simulink model "ava2"  (R2017b)
settings: Solver=VariableStepAuto  StartTime=0.0  StopTime=10.0  RelTol=1e-3
model workspace (MAT data in the model file):
  env_Snm = [1; 1; 1.5; 1.73205080757; 0.866025403784; 2.5; 3.06186217848; 1.9364916731; 0.790569415042; 4.375; 5.53398590529; 3.91311896062; 2.09165006634; 0.739509972887; 7.875; 10.1665812838; 7.68521307447; 4.70621264925; 2.21852991866; 0.70156076002; 14.4375; 18.9031247417; 14.9442322695; 9.96282151301; 5.45686207907; 2.32681380862; 0.671693289381; 26.8125; 35.469603514; 28.960809996; 20.4783851368; 12.3489308748; 6.17446543739; 2.42182459625; 0.647259849288; 50.2734375; 67.03125; 56.0823674036; 41.4195733282; 26.7362196178; 14.8305862683; 6.86522742932; 2.50682661696; 0.62670665424; 94.9609375; 127.403466874; 108.650041615; 82.9828399936; 56.3757383717; 33.6909476871; 17.3979305747; 7.53352492547; 2.58397773171; 0.609049392176; 180.42578125; 243.286073807; 210.691920304; 165.280340459; 116.870849536; 73.9156153223; 41.3200851149; 20.0431853398; 8.18259615041; 2.65478475212; 0.593627917137; 344.44921875; 466.386446929; 409.047973375; 327.968008098; 239.513968234; 158.423598868; 94.1176423013; 49.6043529462; 22.7600380686; 8.81492483989; 2.72034486492; 0.579979473935; 660.194335938; 897.027461585; 795.129860697; 649.220812653; 486.91560949; 334.021352445; 208.298910119; 117.053882271; 58.5269411357; 25.5432512332; 9.43247063627; 2.78148384397; 0.567768012127]
  env_WMMGC = [1 1 2 2 2 3 3 3 3 4 4 4 ... (540 elements, 90x6)]
settings Model: Creator=hbourbou  LastModifiedBy=hbourbou

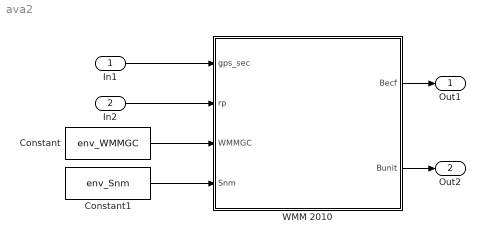
== system ava2 ==
  In1 : Inport
  In2 : Inport  Port=2  PortDimensions=3
  Constant : Constant  Value=env_WMMGC
  Constant1 : Constant  Value=env_Snm
  WMM 2010 : MATLAB Function  TreatAsAtomicUnit=on
  Out1 : Outport
  Out2 : Outport  Port=2
  wires:
  In1/1 -> WMM 2010/1(gps_sec)
  In2/1 -> WMM 2010/2(rp)
  Constant/1 -> WMM 2010/3(WMMGC)
  Constant1/1 -> WMM 2010/4(Snm)
  WMM 2010/1(Becf) -> Out1/1
  WMM 2010/2(Bunit) -> Out2/1

== matlab function ava2/WMM 2010 ==
  data: gps_sec input; Becf output; rp input; WMMGC input; Snm input; Bunit output
%% World Magnetic Model (Valid until Dec 31 2015, needs coefficient update and leap year compesation after this date)
% Requires file magm.m

%% Code
function [Becf, Bunit] = fcn(gps_sec,rp, WMMGC, Snm)


[Becf,Bunit]= magm(rp,gps_sec, WMMGC, Snm);

end

function [Becf,Bunit]=magm(rp,gps_sec,WMMGC, Snm)
%#codegen
% This function computes the magnetic field vector at a given position in space
% Note: altitude limited to 850km above the geomagnetic referemce radius (6371.2 km)

% Vivek Nagabhushan
% May 31 2013le
% Millenium Engineering and Integration Company
% Revised 02/12/2018 Sonny - Model(i.e. WMMGC, snm) is valid through 01/01/2020

% Inputs: Schmidt normalized WMM Gaussian coefficients, position vector in
% the form rp=[phi_gd lambda h_ellp] where, h_ellp is the height above the WGS-84 ellipsoid in kilometers, phi_gd is
% the geodetic latitude in degrees, and lambda is the East longitude from the Greenwich meridian in degrees

% Output: Unit magnetic field vector in ECEF coordinates. Other output forms
% can be chosen if desired

% Other files: index.m, coeffcnvrt.m, R_ECF_NED.m, WMMGC.mat, and Snm.mat

% References:
% 1. Maus, S., S. Macmillan, S. McLean, B. Hamilton, A. Thomson, M. Nair, and C. Rollins, 2010, The US/UK World Magnetic Model for 2010-2015
% 2. Plett, M., 'Magnetic Models' in 'Spacecraft Attitude Determination and Control', Edited by Wertz, J., Kluwer Academic Publishers, 1990
% 3. Davis, J., 'Mathematical Modeling of Earth's Magnetic Field', Technical Note, 'http://hanspeterschaub.info/Papers/UnderGradStudents/MagneticField.pdf', 2004
% 4. Notation for latitude and longitude consistent with Vallado, D. A., 'Fundamentals of Astrodynamics and Applications', 4th Edition, Space Technology Library, 2013

%years since 2015-01-01-00:00:00
% seconds between 2015-01-01-00:00:00 and 1980-01-06:00:00:00 = 1104105616
wmm_sec = gps_sec - 1104105616;
years   = wmm_sec/60/60/24/365;
if(gps_sec > 1140739217) %then leap day has occured!
    years = years + 1/365;
end


r_mag=6371.200; % Geomagnetic reference radius of the Earth in kilometers
Re=6378.137; % Semi-major axis of the Earth ellipsoid / Earth Equatorial radius in kilometers
esquared=0.006694379990141; % Eccentricity that models the Earth oblateness
[g,h]=coeffcnvrt(years, WMMGC, Snm); % Returns Schmidt normalized Gaussian coefficients


phi_gd=rp(1)*pi/180; % Geodetic Latitude
lambda=rp(2)*pi/180; % Geodetic Longitude = Geocentric Longitude
h_ellp=rp(3); % Height above the reference ellipsoid in kilometers (The height reported by GPS is the height above ellipsoid or HAE. The ellipsoid is the WGS84 )

% Convert Geodetic coordinates to Geocentric 
C=Re/sqrt(1-esquared*sin(phi_gd)^2);
rd=(C+h_ellp)*cos(phi_gd);
rk=(C*(1-esquared)+h_ellp)*sin(phi_gd);
r=sqrt(rd^2+rk^2); % Geocentric distance
phi_gc=asin(rk/r); % Conversion from Geodetic Latitude to Geocentric Latitude
co_phi_gc=(pi/2)-phi_gc; % Conversion from latitude to co-latitude
s=sin(co_phi_gc);
c=cos(co_phi_gc);
cl=cos(lambda);
sl=sin(lambda);

K=zeros(90,1);
P=zeros(90,1);
dP=zeros(90,1);
Br=0; 
Bp=0; %B_phi
Bl=0; %B_lambda


% Compute coefficients K and Gaussian-normalized associated Legendre functions, Pnm

P(1)=c;
P(2)=s;
P(3)=c^2-0.33333;
P(4)=c*s;
P(5)=s^2;
dP(1)=-s;
dP(2)=c;
dP(3)=-2*s*c;
dP(4)=c^2-s^2;
dP(5)=2*s*c;


for n=3:12 % Note that values of the fucntions for n=1,2 have been precomputed so that the case of index(0,0) is not encountered
    for m=0:n
        
        if m==n
            P(index(n,m))=s*P(index(n-1,m-1));
            dP(index(n,m))=s*dP(index(n-1,m-1))+c*P(index(n-1,m-1));
        else
            if m>(n-2)
                Pnm2=0;
                dPnm2=0;
            else
                Pnm2=P(index(n-2,m));
                dPnm2=dP(index(n-2,m));
            end
            
            K(index(n,m))=((n-1)^2-m^2)/((2*n-1)*(2*n-3)); % Note that K(1,1) and K(1,0) are equal to zero
            P(index(n,m))=c*P(index(n-1,m))-K(index(n,m))*Pnm2;
            dP(index(n,m))=c*dP(index(n-1,m))-s*P(index(n-1,m))-K(index(n,m))*dPnm2;
        end
               
    end
end


% Spherical coordinate components (Br,B_phi,B_lambda) of magnetic field

cml=0;sml=0;cmm1l=0;smm1l=0; % Initialize to avoid error in Simulink

for n=1:12
    for m=0:n
        
        if m==0
            cml=1; % cos(m*lambda) and sin(m*lambda)
            sml=0; 
            cmm1l=cml; % cos(m-1*(lambda)) and sin((m-1)*lambda) for next iteration
            smm1l=sml; 
        else
            cml=cmm1l*cl-smm1l*sl;
            sml=smm1l*cl+cmm1l*sl;
            cmm1l=cml; % cos(m-1*(phi)) and sin((m-1)*phi) for next iteration
            smm1l=sml; 
        end    
        
        Br=Br+(n+1)*((r_mag/r)^(n+2))*(g(index(n,m))*cml+h(index(n,m))*sml)*P(index(n,m));
        
        Bp=Bp-((r_mag/r)^(n+2))*(g(index(n,m))*cml+h(index(n,m))*sml)*dP(index(n,m));
        
        Bl=Bl-(((r_mag/r)^(n+2))*m*(-g(index(n,m))*sml+h(index(n,m))*cml)*P(index(n,m)))/(s);
        
    end
end

epsilon=phi_gd-phi_gc;

% Earth centric NED coordinates of magnetic field
Bn=-Bp*cos(epsilon)-Br*sin(epsilon); %N
Be=Bl;                               %E
Bd=Bp*sin(epsilon)-Br*cos(epsilon);  %D

Bned=[Bn;Be;Bd];

%Earth centric Earth Fixed (ECEF) components of the magnetic field
Becf=R_ECF_NED(phi_gd,lambda)*Bned;
Bmag=norm(Becf);

Bunit=Becf/Bmag; % Unit magnetic vector in ECEF coordinates
end

function i=index(n,m)
%#codegen
i=0.5*(n*(n+1))+m;

end



function [g,h]=coeffcnvrt(years,WMMGC,Snm)
% This file converts the Schmidt-normalized Gauss coefficients given in the
% NGDC coefficient file to Gaussain coefficients for use in the file magm.m
% Requires the WMM2010 coefficient file by NGDC
% WARNING: This file is valid only till 01 01 2015 00:00:00

% Vivek Nagabhushan
% 06/03/2013
% Millenium Engineering and Integration Company

% Inputs: WMM Coefficient file WWMGC, 
%         time in decimal years (correct to a day)
% Output: Gaussian coefficients 'g' and 'h'

% References:
% 1. Maus, S., S. Macmillan, S. McLean, B. Hamilton, A. Thomson, M. Nair, and C. Rollins, 2010, The US/UK World Magnetic Model for 2010-2015
% 2. Plett, M., 'Magnetic Models' in 'Spacecraft Attitude Determination and Control', Edited by Wertz, J., Kluwer Academic Publishers, 1990
% 3. Davis, J., 'Mathematical Modeling of Earth's Magnetic Field', Technical Note, 'http://hanspeterschaub.info/Papers/UnderGradStudents/MagneticField.pdf', 2004

% End compute decimal years
gmain=WMMGC(1:90,3);
hmain=WMMGC(1:90,4);
gdot=WMMGC(1:90,5);
hdot=WMMGC(1:90,6);

g=Snm.*(gmain+gdot.*years);
h=Snm.*(hmain+hdot.*years);

end



function R=R_ECF_NED(phi_gd,lambda)
%#codegen
%%
%  This function generates the rotation matrix that converts representations in the terrestrial NED coordinate basis to the ECEF frame 
%  The NED basis is formed by: D along the inward normal to the WGS-84 ellipsoid, N along the direction of the North Pole (and E along the Eastward direction)
%  The ECEF bases is formed by: X along the Greenwich meridian in the equatorial plane, Z along the North pole (and Y completes the right-handed system)
%  Input: Geodetic latitude and longitude degrees
%  Output: Rotation matrix from NED to ECEF
%%  References: 
%  1. Vallado, D. A., 'Fundamentals of Astrodynamics and Applications', 4th Edition, Space Technology Library, 2013, pp. 138,144
%  2. World Geodetic System 1984, NIMA TR8350.2, Third Edition, Ammendment 1, Jan 2000, http://earth-info.nga.mil/GandG/publications/tr8350.2/wgs84fin.pdf
%%
%  Vivek Nagabhushan (vnagabhushan@meicompany.com)
%  Millennium Engineering and Integration Company
%  07/02/2013
%%


R=R3(-lambda)*R2((pi/2)+phi_gd);
end

function R=R3(theta)
%#codegen
R=[cos(theta) sin(theta)  0;
  -sin(theta) cos(theta)  0;
       0          0       1];
end

function R=R2(theta)
%#codegen
R=[cos(theta) 0 -sin(theta);
       0      1     0
   sin(theta) 0 cos(theta)];
end
